simulink model "Dynamic_Model"  (R2020b)
settings: Solver=VariableStepAuto  StartTime=0.0  StopTime=300.0  RelTol=1e-3
settings Model: Creator=Obsidian  LastModifiedBy=Obsidian

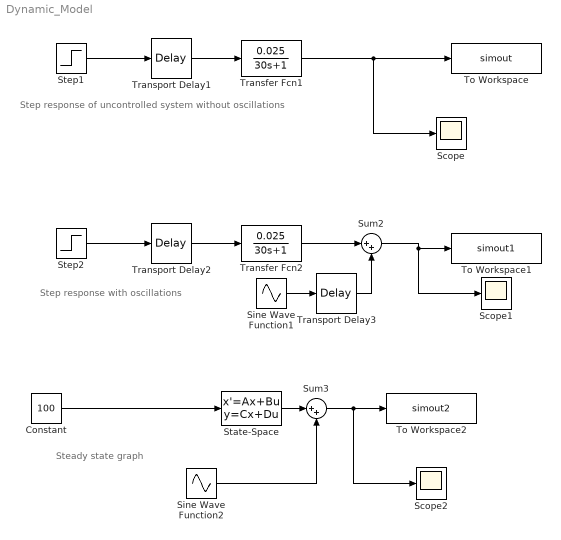
== system Dynamic_Model ==
  note: Step response of uncontrolled system without oscillations
  note: Step response with oscillations
  note: Steady state graph
  Constant : Constant  Value=100
  Scope : Scope
  Scope1 : Scope
  Scope2 : Scope
  Sine Wave Function1 : Sin  Amplitude=0.075  Frequency=10.47  Samples=500  SampleTime=0.01
  Sine Wave Function2 : Sin  Amplitude=0.075  Frequency=10.47  Samples=500  SampleTime=0.01
  State-Space : StateSpace  A=-0.0333  C=8.3333e-04  D=0  InitialCondition=3000
  Step1 : Step  Time=0  After=100  SampleTime=0.01
  Step2 : Step  Time=0  After=100  SampleTime=0.01
  Sum2 : Sum  Inputs=|++
  Sum3 : Sum  Inputs=|++
  To Workspace : ToWorkspace  VariableName=simout  SaveFormat=Structure With Time  SampleTime=-1
  To Workspace1 : ToWorkspace  VariableName=simout1  SaveFormat=Structure With Time  SampleTime=-1
  To Workspace2 : ToWorkspace  VariableName=simout2  SaveFormat=Structure With Time  SampleTime=-1
  Transfer Fcn1 : TransferFcn  Numerator=[0.025]  Denominator=[30 1]
  Transfer Fcn2 : TransferFcn  Numerator=[0.025]  Denominator=[30 1]
  Transport Delay1 : TransportDelay  DelayTime=5
  Transport Delay2 : TransportDelay  DelayTime=5
  Transport Delay3 : TransportDelay  DelayTime=5
  wires:
  Transport Delay1/1 -> Transfer Fcn1/1
  Step1/1 -> Transport Delay1/1
  Transfer Fcn1/1 -> To Workspace/1, Scope/1
  Sine Wave Function1/1 -> Transport Delay3/1
  Transport Delay2/1 -> Transfer Fcn2/1
  Transfer Fcn2/1 -> Sum2/1
  Step2/1 -> Transport Delay2/1
  Sum2/1 -> Scope1/1, To Workspace1/1
  Sum3/1 -> Scope2/1, To Workspace2/1
  State-Space/1 -> Sum3/1
  Sine Wave Function2/1 -> Sum3/2
  Constant/1 -> State-Space/1
  Transport Delay3/1 -> Sum2/2
